simulink model "TestStabilityObserver"  (R2022b)
settings: Solver=FixedStepAuto  StartTime=0.0  StopTime=10.0  FixedStep=simulator.TimeStep  RelTol=1e-3
undefined symbols (not defined in the file): simulator
settings Model: Creator=At  LastModifiedBy=ateay
settings SolverCC: ConcurrentTasks=on  AlgebraicLoopSolver=TrustRegion  InsertRTBMode=Never (minimum delay)
settings DataIOCC: ReturnWorkspaceOutputs=off
settings DebuggingCC: UnconnectedInputMsg=warning  UnconnectedOutputMsg=warning  UnconnectedLineMsg=warning  SFMachineParentedDataDiag=warning  ArithmeticOperatorsInVariantConditions=warning
settings ModelReferenceCC: EnableRefExpFcnMdlSchedulingChecks=on
settings SFSimCC: SimUseLocalCustomCode=off  CustomCodeUndefinedFunction=UseInterfaceOnly
settings RTWCC: RTWUseLocalCustomCode=off
settings CodeAppCC: StateflowObjectComments=on

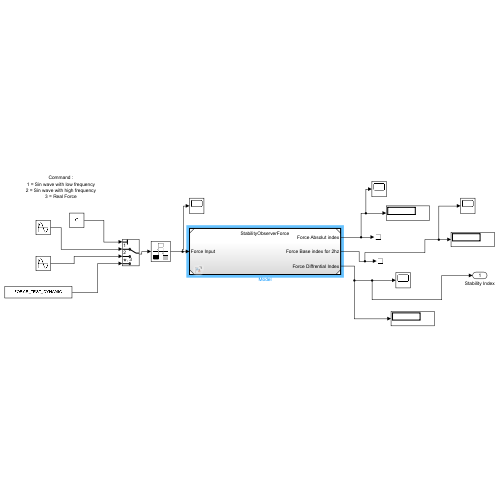
[thumbnail: Simulink's stored preview of the top-level diagram]
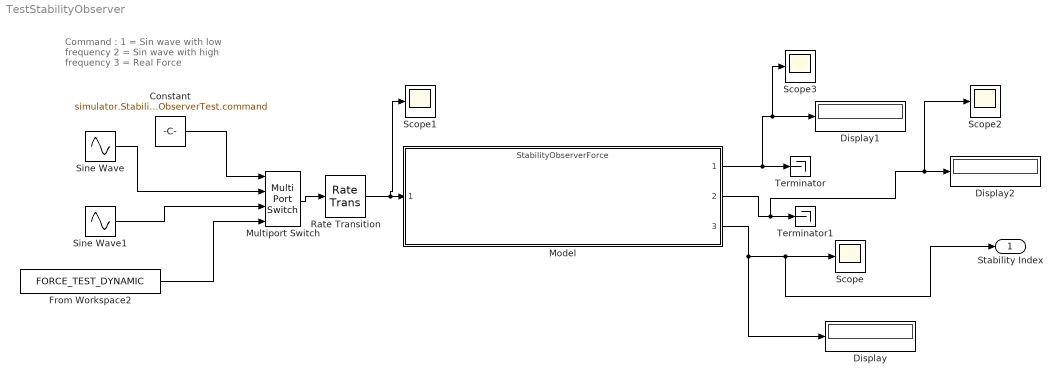
== system TestStabilityObserver ==
  note: Command :
      | 1 = Sin wave with low frequency
      | 2 = Sin wave with high frequency
      | 3 = Real Force
  Constant : Constant  Value=simulator.StabilityObserverTest.command
  Display : Display
      settings: Decimation=5
  Display1 : Display
      settings: Decimation=5
  Display2 : Display
      settings: Decimation=5
  From Workspace2 : FromWorkspace  VariableName=FORCE_TEST_DYNAMIC
  Model : ModelReference  ModelNameDialog=StabilityObserverForce.slx  SimulationMode=Normal  ModelReferenceVersion=1.20
  Multiport Switch : MultiPortSwitch  SaturateOnIntegerOverflow=off  InputSameDT=off
  Rate Transition : RateTransition  Deterministic=off
  Scope{,1..3} (4 alike) : Scope
  Sine Wave : Sin  Amplitude=20  Frequency=2*pi*3  SampleTime=0
  Sine Wave1 : Sin  Amplitude=20  Frequency=2*pi*8  SampleTime=0
  Terminator : Terminator
  Terminator1 : Terminator
  Stability Index : Outport
  wires:
  Model/3 -> Stability Index/1, Scope/1, Display/1
  Model/1 -> Scope3/1, Display1/1, Terminator/1
  Model/2 -> Scope2/1, Display2/1, Terminator1/1
  Rate Transition/1 -> Scope1/1, Model/1
  Constant/1 -> Multiport Switch/1
  Sine Wave/1 -> Multiport Switch/2
  Multiport Switch/1 -> Rate Transition/1
  From Workspace2/1 -> Multiport Switch/4
  Sine Wave1/1 -> Multiport Switch/3
